simulink subsystem "CONTROL_POINTING"  (R2025b)
settings: Solver=VariableStepAuto  StartTime=0.0  StopTime=10.0  RelTol=1e-3
undefined symbols (not defined in the file): tacqAngThres
libraries: simulink x1, aerolibutil x1
settings Model: Creator=antoniohernandez-rodiciomateos  LastModifiedBy=antoniohernandez-rodiciomateos

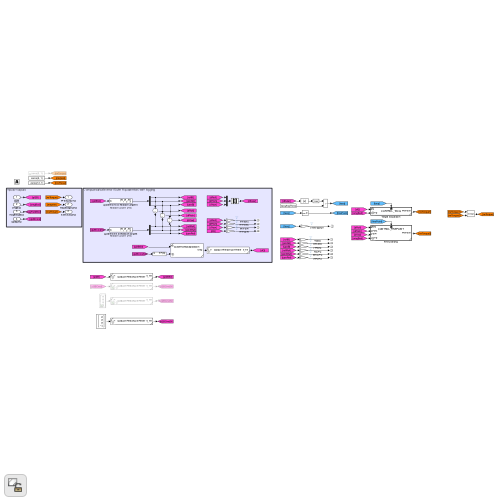
[thumbnail: Simulink's stored preview of the top-level diagram]
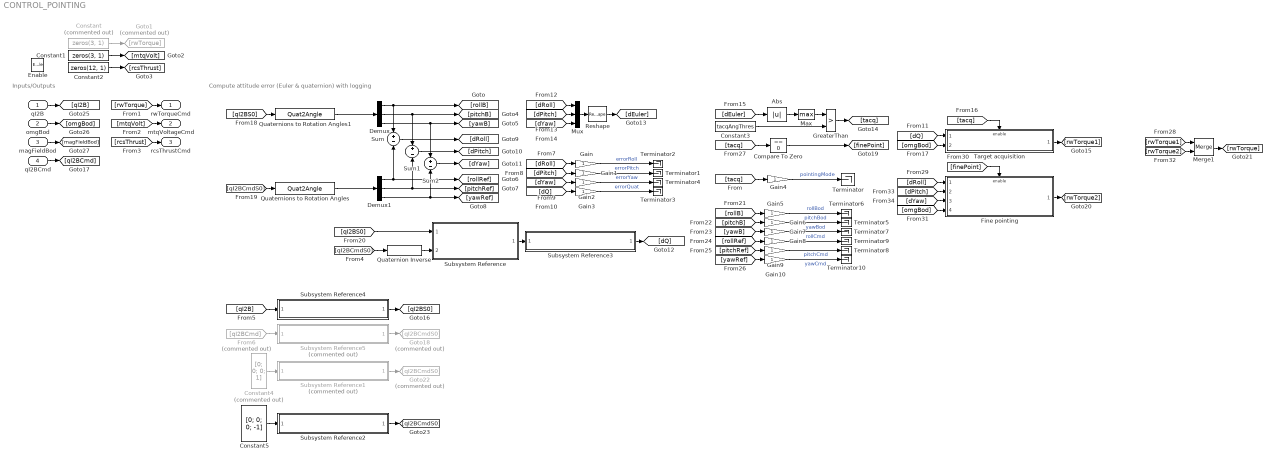
== system CONTROL_POINTING ==
  note: Compute attitude error (Euler & quaternion) with logging
  note: Inputs/Outputs
  qI2B : Inport  OutDataTypeStr=double  PortDimensions=[4 1]
  omgBod : Inport  Port=2  OutDataTypeStr=double  PortDimensions=[3 1]
  magFieldBod : Inport  Port=3  OutDataTypeStr=double  PortDimensions=[3 1]
  qI2BCmd : Inport  Port=4  OutDataTypeStr=double  PortDimensions=[4 1]
  Enable : EnablePort
  Abs : Abs  SaturateOnIntegerOverflow=off
  Compare To Zero : simulink/Logic and Bit Operations/Compare To Zero  relop===  OutDataTypeStr=boolean
  Constant : Constant  Commented=on  Value=zeros(3, 1)
  Constant1 : Constant  Value=zeros(3, 1)
  Constant2 : Constant  Value=zeros(12, 1)
  Constant3 : Constant  Value=tacqAngThres
  Constant4 : Constant  Commented=on  Value=[0; 0; 0; 1]  VectorParams1D=off
  Constant5 : Constant  Value=[0; 0; 0; -1]  VectorParams1D=off
  Demux : Demux  Outputs=3
  Demux1 : Demux  Outputs=3
  Fine pointing : Subsystem  ReferencedSubsystem=CONTROL_FINEPOINT  finePointKp=finePointKp  finePointKd=finePointKd  finePointKn=finePointKn
  From6 : From  Commented=on  GotoTag=qI2BCmd
  Gain{,1..10} (11 alike) : Gain
  Goto1 : Goto  Commented=on  GotoTag=rwTorque
  Goto18 : Goto  Commented=on  GotoTag=qI2BCmdS0
  Goto22 : Goto  Commented=on  GotoTag=qI2BCmdS0
  GreaterThan : RelationalOperator  Operator=>  OutDataTypeStr=boolean  RndMeth=Simplest  InputSameDT=off
  Max : MinMax  Function=max
  Merge1 : Merge
  Mux : Mux  Inputs=3
  Quaternion Inverse : aerolibutil/Quaternion Inverse
  Quaternions to Rotation Angles : Quat2Angle
      settings: AttributesFormatString=Rotation Order: %<rotationOrder>
  Quaternions to Rotation Angles1 : Quat2Angle
      settings: AttributesFormatString=Rotation Order: %<rotationOrder>
  Reshape : Reshape  OutputDimensionality=Column vector (2-D)
  Subsystem Reference : Subsystem  ReferencedSubsystem=quaternionMultiplication  quatMultType=Type 1  quatConv=q0  normQuat=Yes
  Subsystem Reference1 : Subsystem  Commented=on  ReferencedSubsystem=quatConventionConverter  conversion=q4 to q0
  Subsystem Reference2 : Subsystem  ReferencedSubsystem=quatConventionConverter  conversion=q4 to q0
  Subsystem Reference3 : Subsystem  ReferencedSubsystem=quatConventionConverter  conversion=q0 to q4
  Subsystem Reference4 : Subsystem  ReferencedSubsystem=quatConventionConverter  conversion=q4 to q0
  Subsystem Reference5 : Subsystem  Commented=on  ReferencedSubsystem=quatConventionConverter  conversion=q4 to q0
  Sum : Sum  Inputs=+|-
  Sum1 : Sum  Inputs=+|-
  Sum2 : Sum  Inputs=+|-
  Target acquisition : Subsystem  ReferencedSubsystem=CONTROL_TACQ  tacqKp=tacqKp  tacqKd=tacqKd
  Terminator{,1..10} (11 alike) : Terminator
  rwTorqueCmd : Outport  OutDataTypeStr=double  PortDimensions=[3 1]
  mtqVoltageCmd : Outport  Port=2  OutDataTypeStr=double  PortDimensions=[3 1]
  rcsThrustCmd : Outport  Port=3  OutDataTypeStr=double  PortDimensions=[12 1]
  wires:
  [dYaw] -> Fine pointing/3
  [dPitch] -> Fine pointing/2
  [dRoll] -> Fine pointing/1
  [omgBod] -> Fine pointing/4
  [finePoint] -> Fine pointing/Enable
  Fine pointing/1 -> [rwTorque2]
  Merge1/1 -> [rwTorque]
  [rwTorque2] -> Merge1/2
  [rwTorque1] -> Merge1/1
  Compare To Zero/1 -> [finePoint]
  [tacq] -> Compare To Zero/1
  Gain4/1 -> Terminator/1  "pointingMode"
  [yawRef] -> Gain10/1
  [pitchRef] -> Gain9/1
  Gain8/1 -> Terminator9/1  "rollCmd"
  Gain9/1 -> Terminator8/1  "pitchCmd"
  [rollRef] -> Gain8/1
  Gain10/1 -> Terminator10/1  "yawCmd"
  Gain7/1 -> Terminator7/1  "yawBod"
  Gain6/1 -> Terminator5/1  "pitchBod"
  [rollB] -> Gain5/1
  [yawB] -> Gain7/1
  Gain5/1 -> Terminator6/1  "rollBod"
  [pitchB] -> Gain6/1
  [tacq] -> Gain4/1
  Abs/1 -> Max/1
  Max/1 -> GreaterThan/1
  GreaterThan/1 -> [tacq]
  Constant3/1 -> GreaterThan/2
  [dEuler] -> Abs/1
  [qI2BS0] -> Subsystem Reference/1
  [qI2BCmdS0] -> Quaternion Inverse/1
  [qI2BCmdS0] -> Quaternions to Rotation Angles/1
  [qI2BS0] -> Quaternions to Rotation Angles1/1
  [dQ] -> Target acquisition/1
  Target acquisition/1 -> [rwTorque1]
  [tacq] -> Target acquisition/Enable
  [omgBod] -> Target acquisition/2
  Reshape/1 -> [dEuler]
  Mux/1 -> Reshape/1
  [dYaw] -> Mux/3
  [dPitch] -> Mux/2
  [dRoll] -> Mux/1
  Gain3/1 -> Terminator3/1  "errorQuat"
  Gain2/1 -> Terminator4/1  "errorYaw"
  Gain1/1 -> Terminator1/1  "errorPitch"
  Gain/1 -> Terminator2/1  "errorRoll"
  [dQ] -> Gain3/1
  [dYaw] -> Gain2/1
  [dPitch] -> Gain1/1
  [dRoll] -> Gain/1
  Subsystem Reference3/1 -> [dQ]
  Subsystem Reference/1 -> Subsystem Reference3/1
  Quaternion Inverse/1 -> Subsystem Reference/2
  Sum2/1 -> [dYaw]
  Sum1/1 -> [dPitch]
  Sum/1 -> [dRoll]
  Quaternions to Rotation Angles/1 -> Demux1/1
  Demux1/2 -> [pitchRef], Sum1/2
  Demux1/1 -> [rollRef], Sum/2
  Demux1/3 -> [yawRef], Sum2/2
  Quaternions to Rotation Angles1/1 -> Demux/1
  Demux/2 -> [pitchB], Sum1/1
  Demux/1 -> [rollB], Sum/1
  Demux/3 -> [yawB], Sum2/1
  magFieldBod/1 -> [magFieldBod]
  [rwTorque] -> rwTorqueCmd/1
  Constant2/1 -> [rcsThrust]
  Constant1/1 -> [mtqVolt]
  [mtqVolt] -> mtqVoltageCmd/1
  Constant/1 -> Goto1/1
  omgBod/1 -> [omgBod]
  qI2BCmd/1 -> [qI2BCmd]
  [rcsThrust] -> rcsThrustCmd/1
  qI2B/1 -> [qI2B]
  Subsystem Reference1/1 -> Goto22/1
  Subsystem Reference4/1 -> [qI2BS0]
  [qI2B] -> Subsystem Reference4/1
  Subsystem Reference5/1 -> Goto18/1
  Constant4/1 -> Subsystem Reference1/1
  From6/1 -> Subsystem Reference5/1
  Subsystem Reference2/1 -> [qI2BCmdS0]
  Constant5/1 -> Subsystem Reference2/1
